simulink model "controller_stateflow"  (R2022b)
settings: Solver=FixedStepAuto  StartTime=0.0  StopTime=inf  FixedStep=0.05  RelTol=1e-3
PreLoadFcn:
  | rosinit();
model workspace (MAT data in the model file):
  SL_ROS_VariableLengthArrays_MaxSizes : object (value not decoded)
  pitch = -10
  restart = 0
undefined symbols (not defined in the file): StartTime
libraries: robotmaniplib x62, robotlib x17, robotcorelib x4, robotgazebolib x1
(part 3 of 4)

== matlab function controller_stateflow/Panda Controller Command/panda_TrajectoryController_command ==
  data: Time input; msgOut output Bus: SL_Bus_controller_stateflow_trajectory_msgs_JointTrajectory; msgIn input; msgPoint input; TimeFromStart input; Point_array input
function msgOut   = panda_TrajectoryController_command(Time, msgIn, msgPoint, TimeFromStart, Point_array)
% In this function we create the TrajecotryJointController message for the
% ROS topic to command movements of manipulator.
    msgOut = msgIn;
    if Time.Sec ~= 0

        jointNames = {'panda_joint1','panda_joint2','panda_joint3'...
            'panda_joint4','panda_joint5','panda_joint6','panda_joint7'};
        numJoints = uint32(length(jointNames));
        msgOut.JointNames_SL_Info.CurrentLength = numJoints;
        for idx = 1:numJoints
            jName = jointNames{idx};
            lenName = uint32(length(jName));
            msgOut.JointNames(idx).Data(1:lenName) = uint8(jName);
            msgOut.JointNames(idx).Data_SL_Info.CurrentLength = lenName;
        end
        
        msgOut.Header.Stamp.Sec = Time.Sec;
        msgOut.Header.Stamp.Nsec = Time.Nsec;
        
        msgOut.Header.Seq = uint32(0);

        %if the points are all equals, the command is to reach that point
        %in one pooint position command, in TimeFromStart time.
        if isequal(Point_array(:,1),Point_array(:,2))
            msgOut.Points_SL_Info.CurrentLength = uint32(1);
            msgOut.Points(1) = msgPoint;
            msgOut.Points(1).Positions(1:7) = Point_array(1:7,1);
            msgOut.Points(1).Positions_SL_Info.CurrentLength = uint32(7);
            msgOut.Points(1).TimeFromStart.Sec = TimeFromStart;
            msgOut.Points(1).TimeFromStart.Nsec = 0;
        else
            % otherwise the command is a trajectory command and the time is
            % divided for each point.
            msgOut.Points_SL_Info.CurrentLength = uint32(size(Point_array,2));
    
            for i = 1:size(Point_array,2)
                msgOut.Points(i) = msgPoint;
                msgOut.Points(i).Positions(1:7) = Point_array(1:7,i);
                msgOut.Points(i).Positions_SL_Info.CurrentLength = uint32(7);
       
                time = TimeFromStart*1e9;
                time_i_nsec = time/5*i;
                msgOut.Points(i).TimeFromStart.Sec = fix(time_i_nsec/1e9);
                msgOut.Points(i).TimeFromStart.Nsec = time_i_nsec-fix(time_i_nsec/1e9);
            end
        end

    end
end

== stateflow chart controller_stateflow/Chart ==
  state wait_command
    enable = 0;
    finish_ur=0;
  state send
    enable = 1;
  state wait
    enable = 0;
  state succes
    finish_ur=1;
  (default) -> wait_command
  send -> wait
  wait_command -> send : [command == 1]
  wait -> succes : [ok == 1]
  succes -> wait_command : [command == 0]
  data: enable output; ok input; finish_ur output; command input

== matlab function controller_stateflow/Summit Controller Command/summit_VelocityController_command ==
  data: Time input; msgOut output Bus: SL_Bus_controller_stateflow_geometry_msgs_Twist; msgIn input; sum_cntr input
function msgOut   = summit_VelocityController_command(Time, msgIn, sum_cntr)
% This function populates the message to command summit pose

    msgOut = msgIn;
    if Time.Sec ~= 0
            msgOut.Linear.X = sum_cntr(1);
            msgOut.Linear.Y = sum_cntr(2);
            msgOut.Linear.Z = 0;
            msgOut.Angular.X = 0;
            msgOut.Angular.Y = 0;
            msgOut.Angular.Z = sum_cntr(3);
    end
end

== matlab function controller_stateflow/UR10e compare ==
  data: goal_ input size=[6,5]; actual input; ok output; tol input
function ok = compare(goal_, actual,tol)
% This function compare the actual and desired position with a tolerance

    goal = zeros(6,1);
    goal = goal_(:,5);
    ok = 0;
    
    if  actual(1) <= goal(1) + tol && actual(1) >= goal(1) - tol && ...
        actual(2) <= goal(2) + tol && actual(2) >= goal(2) - tol && ...
        actual(3) <= goal(3) + tol && actual(3) >= goal(3) - tol && ...
        actual(4) <= goal(4) + tol && actual(4) >= goal(4) - tol && ...
        actual(5) <= goal(5) + tol && actual(5) >= goal(5) - tol && ...
        actual(6) <= goal(6) + tol && actual(6) >= goal(6) - tol 
        
        ok=1;
    end
end

== stateflow chart controller_stateflow/Chart1 ==
  state wait_command
    enable = 0;
    finish_panda=0;
  state send
    enable = 1;
  state wait
    enable = 0;
  state succes
    finish_panda=1;
  (default) -> wait_command
  send -> wait
  wait_command -> send : [command == 1]
  wait -> succes : [ok == 1]
  succes -> wait_command : [command == 0]
  data: enable output; ok input; command input; finish_panda output

== matlab function controller_stateflow/Panda compare ==
  data: goal_ input size=[7,5]; actual input; ok output; tol input
function ok = compare(goal_, actual,tol)
% This function compare the actual and desired position with a tolerance

    goal = zeros(7,1);
    goal = goal_(:,5);
    ok = 0;
    
    if  actual(1) <= goal(1) + tol && actual(1) >= goal(1) - tol && ...
        actual(2) <= goal(2) + tol && actual(2) >= goal(2) - tol && ...
        actual(3) <= goal(3) + tol && actual(3) >= goal(3) - tol && ...
        actual(4) <= goal(4) + tol && actual(4) >= goal(4) - tol && ...
        actual(5) <= goal(5) + tol && actual(5) >= goal(5) - tol && ...
        actual(6) <= goal(6) + tol && actual(6) >= goal(6) - tol && ...
        actual(7) <= goal(7) + tol && actual(7) >= goal(7) - tol
        ok=1;
    end

end

== stateflow chart controller_stateflow/Chart2 ==
  state wait_command
    finish_sum=0;
  state wait
  state succes
    finish_sum=1;
  (default) -> wait_command
  wait_command -> wait : [command == 1]
  wait -> succes : [ok == 1]
  succes -> wait_command : [command==0]
  data: finish_sum output; ok input; command input

== matlab function controller_stateflow/General State Flow/get_ur_pose_cnvy/MATLAB Function1 ==
  data: Pose output; traPos input; traZYX input; sumPos input; sumZYX input; urState input; Weights output; initialGuess output; state input; NWayPoints output; durTime output
function [Pose, Weights, initialGuess ,NWayPoints,durTime] = fcn(traPos,traZYX,sumPos,sumZYX,urState,state)

traDim = [1;5.456930;0.192575];

% back_from_box = traPos + [eul2rotm(tra_ZYX', 'ZYX')]*[0; traDim(2)/2 + +0.7+distance_xx + base_sum_length/2;0];

toSumChapa = [0;0;0.51];
toUR10e = [0.35;0.32+0.04;0.05];
base_ur_offset = [0;0;0.035];

traPos_offset = [0;0;0];

NWayPoints = 1;
durTime = 2;
distance = eye(4,4);
ZYX_d = [0,0,0];

if state == 1
    traPos_offset = [0; traDim(2)/2 + 0.0;traDim(3)/2+0.03];
    NWayPoints = 1;
    durTime = 2;
end


traPos0 = traPos+[eul2rotm(traZYX', 'ZYX')]*traPos_offset;

% trasformazione world -> box::frame
% boxtf_01 = [[eul2rotm(boxZYX', 'ZYX')],boxPos; ...
%             0 0 0                               1           ];

% Trasformazione world -> summit::base_footprint
sumtf_01 = [[eul2rotm(sumZYX', 'ZYX')],sumPos; ...
            0 0 0                               1           ];
% Trasformazione summit::base_footprint -> UR10e::base
sumtoUR10etf_12 = [[eul2rotm([0,0,0], 'ZYX')],toSumChapa+toUR10e+base_ur_offset; ...
            0 0 0                               1           ];
% Trasformazione world -> UR10e::base
toUR10etf = sumtf_01*sumtoUR10etf_12;

% Trasformo la posa da world frame a UR10e::base frame per l'IK
% Point_d0 = boxtf_01*[[eul2rotm(ZYX_d,'ZYX')],[boxPos_offset(1);boxPos_offset(2);boxPos_offset(3)]; ...
%                                 0 0 0                               1           ];
% 
% Pose = distance*inv(toUR10etf)*Point_d0;

tra_ = inv(toUR10etf)*[traPos0;1];

Pose = [[eul2rotm(ZYX_d,'ZYX')],[tra_(1);tra_(2);tra_(3)]; ...
            0 0 0                               1           ];

Weights = [1,1,1,1,1,1];
initialGuess = urState(1:6,1);


end

== matlab function controller_stateflow/summit_control ==
  data: goal_position input double size=[3,1]; goal_orientationZYX input double size=[3,1]; pose input; orientationZYX input; ok output double size=[1,1]; tol_p input; sum_cntr output; tol_or input
function [ok,sum_cntr] = summit_control(goal_position, goal_orientationZYX,pose,orientationZYX,tol_p,tol_or)
% This function compare the actual and the desired position and orientation
% of the mobile robot and compute the control to reach goals.

    ok = 0;
    if  pose(1) <= goal_position(1) + tol_p && pose(1) >= goal_position(1) - tol_p && ...
        pose(2) <= goal_position(2) + tol_p && pose(2) >= goal_position(2) - tol_p && ...
        orientationZYX(1) <= goal_orientationZYX(1) + tol_or && orientationZYX(1) >= goal_orientationZYX(1) - tol_or
       
        ok=1;
    end
    
    % Compute the control command for the velocity controller in
    % ROS Planar Move Plugin
    k = 0.5;
    theta = orientationZYX(1);
    e_X = k*(goal_position(1)- pose(1));
    e_Y = k*(goal_position(2)- pose(2));

    cntr_posX = e_X*cos(theta)+e_Y*sin(theta);
    cntr_posY = -e_X*sin(theta)+e_Y*cos(theta);

    cntr_orZ  = k*(goal_orientationZYX(1)- orientationZYX(1));
    
    sum_cntr = [cntr_posX,cntr_posY,cntr_orZ];

end

== matlab function controller_stateflow/General State Flow/get_ur_pose/MATLAB Function ==
  data: Pose output; boxPos input; boxZYX input; sumPos input; sumZYX input; urState input; Weights output; initialGuess output; state input; NWayPoints output; durTime output
function [Pose, Weights, initialGuess, NWayPoints, durTime] = fcn(boxPos,boxZYX,sumPos,sumZYX,urState,state)

distance_10 = 0.2;
dimBox=[0.38,0.18,0.14];
toSumChapa = [0;0;0.51];
toUR10e = [0.35;0.32+0.02;0.05];
base_ur_offset = [0;0;0.035];

NWayPoints = 1;
durTime = 2;
distance = eye(4,4);
boxPos_offset = [0;0;0];
ZYX_d = [0,0,0];

% in base allo stato in cui si trovano, definisco punto in cui deve andare
% l'end-effector relativamente alla scatola,l'orientazione dell'ee, la 
% distanza da tale punto, il modo e il tempo
if state == 2
    boxPos_offset = [0;-dimBox(2)/2;-dimBox(3)/2];
    ZYX_d = [pi/2,0,0];
    distance = [[eul2rotm([0,0,0],'ZYX')],[-distance_10,0,0]'; ...
                       0 0 0              1   ];
    NWayPoints = 1;
    durTime = 2;
end

if state == 4
    boxPos_offset = [0;-dimBox(2)/2;-dimBox(3)/2];
    ZYX_d = [pi/2,0,0];
    NWayPoints = 1;
    durTime = 2;
end

% if state == 11
%     boxPos_offset = [0;-dimBox(2)/2;-dimBox(3)/2];
%     ZYX_d = [pi/2,0,0];
%     NWayPoints = 1;
%     durTime = 2;
% end
% 
% if state == 12
%     boxPos_offset = [0;-dimBox(2)/2;-dimBox(3)/2];
%     ZYX_d = [pi/2,0,0];
%     NWayPoints = 1;
%     durTime = 2;
% end

if state == 7
    boxPos_offset = [0;+dimBox(2)/2;-dimBox(3)/2];
    ZYX_d = [pi/2,0,0];
    boxPos =[1;0;0.65];     %pose in terna summit::base_footprint
    boxZYX =[-pi/2;0;0];
    sumPos = [0;0;0];
    sumZYX = [0;0;0];
    NWayPoints = 5;
    durTime = 4;
end


% trasformazione world -> box::frame
boxtf_01 = [[eul2rotm(boxZYX', 'ZYX')],boxPos; ...
            0 0 0                               1           ];

% Trasformazione world -> summit::base_footprint
sumtf_01 = [[eul2rotm(sumZYX', 'ZYX')],sumPos; ...
            0 0 0                               1           ];
% Trasformazione summit::base_footprint -> UR10e::base
sumtoUR10etf_12 = [[eul2rotm([0,0,0], 'ZYX')],toSumChapa+toUR10e+base_ur_offset; ...
            0 0 0                               1           ];
% Trasformazione world -> UR10e::base
toUR10etf = sumtf_01*sumtoUR10etf_12;

% Trasformo la posa da world frame a UR10e::base frame per l'IK
Point_d0 = boxtf_01*[[eul2rotm(ZYX_d,'ZYX')],[boxPos_offset(1);boxPos_offset(2);boxPos_offset(3)]; ...
                                0 0 0                               1           ];

Pose = distance*inv(toUR10etf)*Point_d0;

Weights = [1,1,1,1,1,1];
initialGuess = urState(1:6,1);

end

== matlab function controller_stateflow/General State Flow/get_ur_pose_cnvy/MATLAB Function2 ==
  data: pose_d input; Pose1 output; T input; Pose2 output; Pose3 output; NWayPoint input; Pose4 output; Pose5 output
function [Pose1,Pose2,Pose3,Pose4,Pose5] = fcn(pose_d,T,NWayPoint)

    coder.extrinsic('slerp');

    if NWayPoint == 1
        Pose1 = pose_d;
        Pose2 = pose_d;
        Pose3 = pose_d;
        Pose4 = pose_d;
        Pose5 = pose_d;
    else

        %semplice interpolazione lineare sulla posizione tra posizione
        %attuale e posizione desiderata
        pos_act   = T(1:3,4);
        pos_d     = pose_d(1:3,4);
        delta_pos = (pos_d-pos_act)/5; 
                  
        q_d = rotm2quat(pose_d(1:3,1:3));
        q_a = rotm2quat(T(1:3,1:3));
        q =   slerp(quaternion(q_a),quaternion(q_d),0:0.2:1);

        Pose1 = [quat2rotm(q(1)),pos_act+delta_pos*1; ...
                 0 0 0                               1           ];
        Pose2 = [quat2rotm(q(2)),pos_act+delta_pos*2; ...
                 0 0 0                               1           ];
        Pose3 = [quat2rotm(q(3)),pos_act+delta_pos*3; ...
                 0 0 0                               1           ];
        Pose4 = [quat2rotm(q(4)),pos_act+delta_pos*4; ...
                 0 0 0                               1           ];

        Pose5 = pose_d;
    end

end

== matlab function controller_stateflow/Subsystem6/MATLAB Function8 ==
  data: pick_type input; box1 output Bus: SL_Bus_controller_stateflow_geometry_msgs_Pose; box2 output Bus: SL_Bus_controller_stateflow_geometry_msgs_Pose; link_states input; sum_pose output Bus: SL_Bus_controller_stateflow_geometry_msgs_Pose; pose input Bus: SL_Bus_controller_stateflow_geometry_msgs_Pose; conveyorbelt output Bus: SL_Bus_controller_stateflow_geometry_msgs_Pose
function [box1,box2,sum_pose,conveyorbelt] = link_state_subscriber(pick_type, link_states, pose)
    
    % Initialize function parameters
    sum_pose=pose;
    idx_sum = 0;
    box1 = pose;
    box2 = pose;
    idx_box1 = 0;
    idx_box2 = 0;
    conveyorbelt = pose;
    idx_tra = 0;

    % Set the right box name based on the type of picking primitive
    box_string  = 'box_38_18_14::link_0';
    box_string2 = 'box_38_18_14_0::link_0';
    if pick_type == 2
        box_string = 'box_19_14_29::link_0';
        else if pick_type == 3
                    box_string = 'cilinder_20_13::link_0';
        end
    end

    % Get links info by link_states message from Gazebo Publisher
    linkName = uint32(length(link_states.Name));
    for i = 1:linkName
        link = char(link_states.Name(i).Data');
        link_ = deblank(link);
        if strcmp(link_,'iliad::summitxls_base_footprint')
            idx_sum = double(i);
        end
        if strcmp(link_,box_string)  % type 3    
            idx_box1 = double(i);
        end
        if (pick_type == 4 && strcmp(link_,box_string2))  % type 4    
            idx_box2 = double(i);
        end
        if strcmp(link_,'transporter::link_0')
            idx_tra = double(i);
        end

    end

    sum_pose = link_states.Pose(idx_sum);
    box1 = link_states.Pose(idx_box1);    
    conveyorbelt = link_states.Pose(idx_tra);
    
    % if we are not in case 4, set the second box pose equal to the first
    % one
    if (pick_type == 4)
        box2 = link_states.Pose(idx_box2);
    else
        box2 = link_states.Pose(idx_box1);
    end

end

== matlab function controller_stateflow/General State Flow/get_panda_pose/MATLAB Function ==
  data: Pose output; boxPos input; boxZYX input; sumPos input; sumZYX input; panda_state input; Weights output; initialGuess output; state input; NWayPoints output; durTime output
function [Pose, Weights, initialGuess, NWayPoints, durTime] = fcn(boxPos,boxZYX,sumPos,sumZYX,panda_state,state)
    
    distance_10 = 0.2;
    distance_10_h = 0.1;
    dimBox=[0.38,0.18,0.14];
    toSumChapa = [0;0;0.51];
    toFranka = [0.25;-0.22+0.02;0.15];
    boxPos_offset = [0;0;0];
    
    NWayPoints = 1;
    durTime = 2;
    distance = eye(4,4);
    ZYX_d = [0,0,0];

    Weights = [1,1,1,1,1,1];


    if state == 2
        boxPos_offset = [-0.02;dimBox(2)/2+0.02;+dimBox(3)/2];
        ZYX_d = [pi+pi/2,-pi/4,0];
        distance = [[eul2rotm([0,0,0],'ZYX')],[-distance_10,0,distance_10_h]'; ...
                                0 0 0                       1              ];
        NWayPoints = 1;
        durTime = 2;
    end

    if state == 4
        boxPos_offset = [-0.02;dimBox(2)/2+0.015;dimBox(3)/2-0.05];
        ZYX_d = [pi+pi/2,-pi/4,0];
        NWayPoints = 1;
        durTime = 2;
    end
    if state == 5
        boxPos_offset = [-0.02;-dimBox(2)/2+0.04;+dimBox(3)/2-0.05];
        ZYX_d = [pi+pi/2,-pi/4,0];
        NWayPoints = 1;
        durTime = 2;
    end
    if state == 122
        boxPos_offset = [-0.02;dimBox(2)/2+0.04;dimBox(3)/2-0.05];
        ZYX_d = [pi+pi/2,-pi/8,0];
        NWayPoints = 1;
        durTime = 2;
    end

    if state == 6
        boxPos_offset = [-0.02;dimBox(2)/2+0.04;dimBox(3)/2-0.03];
        ZYX_d = [pi+pi/2,-pi/16,0];
        NWayPoints = 1;
        durTime = 2;
    end

    if state == 7
        boxPos_offset = [-0.02;dimBox(2)/2+0.04;dimBox(3)/2-0.03];
        ZYX_d = [pi+pi/2,-pi/16,0];
        boxPos =[1;0;0.65];     %pose in terna summit::base_footprint
        boxZYX =[-pi/2;0;0];
        sumPos = [0;0;0];
        sumZYX = [0;0;0];
        NWayPoints = 5;
        durTime = 4;
    end

    if state == 93
        boxPos_offset = [0;0.05;0.35+dimBox(3)/2];
        ZYX_d = [pi+pi/2,-pi/4,0];
        NWayPoints = 1;
        durTime = 2;
    end
    
    % Trasformazione world -> box::frame
    boxtf_01 = [[eul2rotm(boxZYX', 'ZYX')],boxPos; ...
            0 0 0                               1           ];
    % Trasformazione world -> summit::base_footprint
    sumtf_01 = [[eul2rotm(sumZYX', 'ZYX')],sumPos; ...
                0 0 0                               1           ];
    
    % Trasformazione summit::base_footprint -> panda::base
    sumtopandatf_12 = [[eul2rotm([0,pi/4,0], 'ZYX')],toSumChapa+toFranka; ...
                0 0 0                               1           ];
    
    % Trasformazione world -> panda::base
    toPandatf = sumtf_01*sumtopandatf_12;
    
    % Trasformo la posizione da world frame a panda::base frame per l'IK
    Pose_d0 = boxtf_01*[[eul2rotm(ZYX_d,'ZYX')],[boxPos_offset(1);boxPos_offset(2);boxPos_offset(3)]; ...
                                0 0 0                               1           ];

    Pose = distance*inv(toPandatf)*Pose_d0;

    initialGuess = panda_state;
    
    if state == 2
         initialGuess = [0;-0.7853;0;-2.35619;0;1.57079;0.785398];

    end

end
